simulink subsystem "model_inductance_L1"  (R2024a)
settings: Solver=VariableStepAuto  StartTime=0.0  StopTime=10.0  RelTol=1e-3
settings Model: Creator=Bocchio  LastModifiedBy=Bocchio

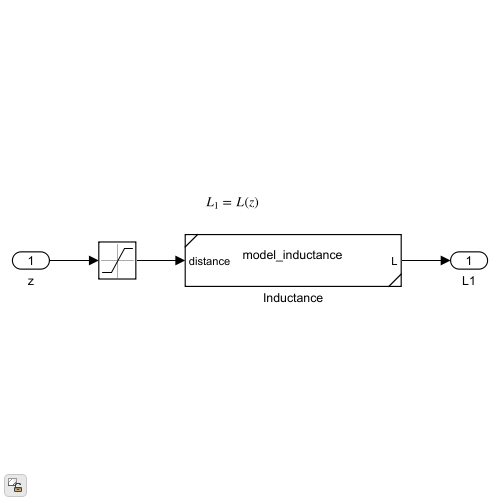
[thumbnail: Simulink's stored preview of the top-level diagram]
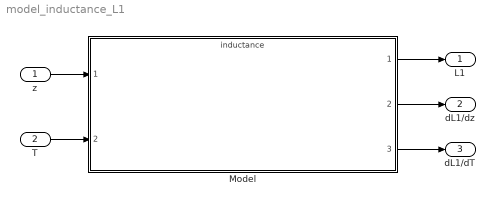
== system model_inductance_L1 ==
  z : Inport
  T : Inport  Port=2
  Model : ModelReference  ModelNameDialog=inductance.slx  SimulationMode=Normal  ModelReferenceVersion=1.2
  L1 : Outport
  dL1/dz : Outport  Port=2
  dL1/dT : Outport  Port=3
  wires:
  Model/3 -> dL1/dT/1
  Model/2 -> dL1/dz/1
  Model/1 -> L1/1
  z/1 -> Model/1
  T/1 -> Model/2
